simulink model "Step"  (R2020a)
settings: Solver=VariableStepAuto  StartTime=0.0  StopTime=0.75  RelTol=1e-3
settings Model: Creator=João Fernando Rangel  LastModifiedBy=João Fernando Rangel

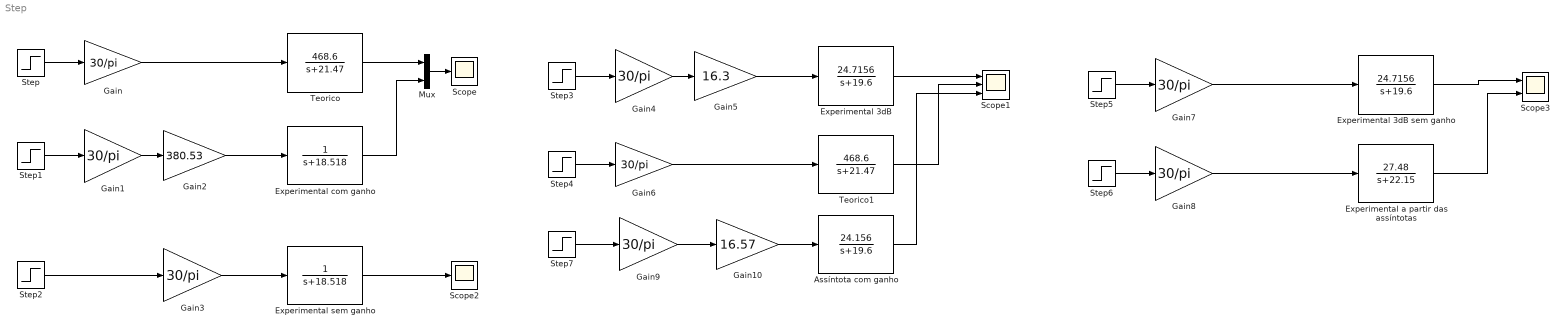
== system Step ==
  Assíntota com ganho : TransferFcn  Numerator=[24.156]  Denominator=[1 19.6]
  Experimental 3dB : TransferFcn  Numerator=[24.7156]  Denominator=[1 19.6]
  "Experimental 3dB sem ganho " : TransferFcn  Numerator=[24.7156]  Denominator=[1 19.6]
  Experimental a partir das assíntotas : TransferFcn  Numerator=[27.48]  Denominator=[1 22.15]
  Experimental com ganho : TransferFcn  Denominator=[1 18.518]
  Experimental sem ganho : TransferFcn  Denominator=[1 18.518]
  Gain{,1,3..4,6..9} (8 alike) : Gain  Gain=30/pi
  Gain10 : Gain  Gain=16.57
  Gain2 : Gain  Gain=380.53
  Gain5 : Gain  Gain=16.3
  Mux : Mux  Inputs=2
  Scope : Scope
  Scope1 : Scope  NumInputPorts=3
  Scope2 : Scope
  Scope3 : Scope  NumInputPorts=2
  Step{,1,3..4,7} (5 alike) : Step  Time=0.1  After=24  SampleTime=0
  Step2 : Step  Time=0  After=24  SampleTime=0
  Step5 : Step  Time=0  After=24  SampleTime=0
  Step6 : Step  Time=0  After=24  SampleTime=0
  Teorico : TransferFcn  Numerator=[468.6]  Denominator=[1 21.47]
  Teorico1 : TransferFcn  Numerator=[468.6]  Denominator=[1 21.47]
  wires:
  Step/1 -> Gain/1
  Gain/1 -> Teorico/1
  Gain1/1 -> Gain2/1
  Step1/1 -> Gain1/1
  Teorico/1 -> Mux/1
  Mux/1 -> Scope/1
  Gain2/1 -> Experimental com ganho/1
  Experimental com ganho/1 -> Mux/2
  Step2/1 -> Gain3/1
  Gain3/1 -> Experimental sem ganho/1
  Experimental sem ganho/1 -> Scope2/1
  Gain4/1 -> Gain5/1
  Step3/1 -> Gain4/1
  Gain5/1 -> Experimental 3dB/1
  Teorico1/1 -> Scope1/2
  Gain6/1 -> Teorico1/1
  Step4/1 -> Gain6/1
  Experimental 3dB/1 -> Scope1/1
  Gain7/1 -> "Experimental 3dB sem ganho "/1
  Step5/1 -> Gain7/1
  "Experimental 3dB sem ganho "/1 -> Scope3/1
  Experimental a partir das assíntotas/1 -> Scope3/2
  Step6/1 -> Gain8/1
  Gain8/1 -> Experimental a partir das assíntotas/1
  Gain9/1 -> Gain10/1
  Step7/1 -> Gain9/1
  Assíntota com ganho/1 -> Scope1/3
  Gain10/1 -> Assíntota com ganho/1
